simulink model "MPU_Test9250_ArduinoSerialb"  (R2020b)
settings: Solver=FixedStepDiscrete  StartTime=0.0  StopTime=inf  FixedStep=0.02  RelTol=1e-3  EnableMultiTasking=on
libraries: arduinosensorlib x2, etargetslib x2, arduinolib x2
settings Model: SILPILModeSetting=veronly  EnablePacing=on  ExtModeTrigDuration=2  Creator=eber_  LastModifiedBy=eber_
settings OptimizationCC: EnhancedBackFolding=on  PassReuseOutputArgsAs=Individual arguments  ZeroExternalMemoryAtStartup=off  ZeroInternalMemoryAtStartup=off  MaxStackSize=64  OptimizeBlockOrder=speed  DifferentSizesBufferReuse=on  OptimizationCustomize=off  EfficientTunableParamExpr=on
settings DebuggingCC: ParameterTunabilityLossMsg=error
settings HardwareCC: ProdBitPerInt=16  ProdBitPerPointer=16  ProdBitPerSizeT=16  ProdBitPerPtrDiffT=16  ProdLargestAtomicFloat=None  ProdWordSize=8  ProdHWDeviceType=Atmel->AVR
settings SFSimCC: MATLABDynamicMemAlloc=off
settings RTWCC: Description=Embedded Coder  SystemTargetFile=ert.tlc  HardwareBoard=Arduino Nano 3.0  TemplateMakefile=ert_default_tmf  Toolchain=Arduino AVR  BuildConfiguration=Faster Runs
settings CodeAppCC: ForceParamTrailComments=on  IgnoreCustomStorageClasses=off  OperatorAnnotations=on  SimulinkDataObjDesc=on  SFDataObjDesc=on  InsertBlockDesc=on
settings ERTTargetCC: SupportContinuousTime=on  SupportVariableSizeSignals=on  ExtModeStaticAllocSize=250

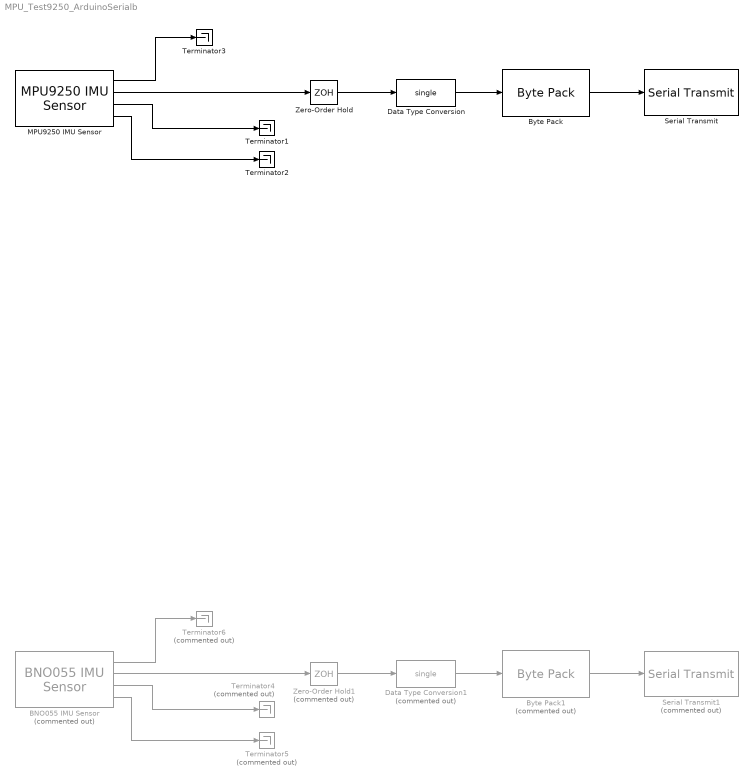
== system MPU_Test9250_ArduinoSerialb ==
  BNO055 IMU Sensor : arduinosensorlib/BNO055 IMU Sensor  Commented=on  SlaveAddress=0x28  OperationMode=Fusion  Accel=on  AngularRate=on  MagField=on  EulerAngles=off  Quat=off  LinearAccel=off  GravityVector=off  AccelRange=4G  AccelBW=62.5 Hz  GyroRange=2000 dps  GyroBW=32 Hz  MagODR=10 Hz  SampleTime=0.0125  blockPlatform=ARDUINO
      settings: SourceProductBaseCode=ARDUINO
  Byte Pack : etargetslib/Byte Pack  datatypes={'single'}  byteAlign=4
  Byte Pack1 : etargetslib/Byte Pack  Commented=on  datatypes={'single'}  byteAlign=4
  Data Type Conversion : DataTypeConversion  OutDataTypeStr=single
  Data Type Conversion1 : DataTypeConversion  Commented=on  OutDataTypeStr=single
  MPU9250 IMU Sensor : arduinosensorlib/MPU9250 IMU Sensor  SlaveAddress=0x68  Accel=on  AngularRate=on  Ak8963Field=on  Temperature=on  Status=off  EulerAngles=off  Quat=off  AccelRange=2G  Acceldlpf=218.1 Hz  GyroRange=250 dps  Gyrodlpf=250 Hz  DmpOdr=200 Hz  SampleTime=-1
      settings: SourceProductBaseCode=ARDUINO
  Serial Transmit : arduinolib/Serial Transmit  portNumber=0  sendmode=write  sendformat=Decimal  floatprecision=2  blockPlatform=arduino
  Serial Transmit1 : arduinolib/Serial Transmit  Commented=on  portNumber=0  sendmode=write  sendformat=Decimal  floatprecision=2  blockPlatform=arduino
  Terminator1 : Terminator
  Terminator2 : Terminator
  Terminator3 : Terminator
  Terminator4 : Terminator  Commented=on
  Terminator5 : Terminator  Commented=on
  Terminator6 : Terminator  Commented=on
  Zero-Order Hold : ZeroOrderHold  SampleTime=-1
  Zero-Order Hold1 : ZeroOrderHold  Commented=on  SampleTime=-1
  wires:
  MPU9250 IMU Sensor/2 -> Zero-Order Hold/1
  MPU9250 IMU Sensor/3 -> Terminator1/1
  MPU9250 IMU Sensor/4 -> Terminator2/1
  Zero-Order Hold/1 -> Data Type Conversion/1
  Data Type Conversion/1 -> Byte Pack/1
  Byte Pack/1 -> Serial Transmit/1
  MPU9250 IMU Sensor/1 -> Terminator3/1
  BNO055 IMU Sensor/1 -> Terminator6/1
  Byte Pack1/1 -> Serial Transmit1/1
  Data Type Conversion1/1 -> Byte Pack1/1
  Zero-Order Hold1/1 -> Data Type Conversion1/1
  BNO055 IMU Sensor/4 -> Terminator5/1
  BNO055 IMU Sensor/3 -> Terminator4/1
  BNO055 IMU Sensor/2 -> Zero-Order Hold1/1
